simulink model "gm_HDL_pfc_gold_fi_og"  (R2024b)
settings: Solver=FixedStepDiscrete  StartTime=0.0  StopTime=.2  RelTol=1e-3
InitFcn:
  | fidelity_pfc_vals;
  | nbits=(2^12)-2;
  | A_mat = fi(stateSpaceParameters_1.Ad,1,25,24);
  | B_mat = fi(stateSpaceParameters_1.Bd,1,25,31);
  | C_mat = fi(stateSpaceParameters_1.Cd,1,25,20);
  | D_mat = fi(stateSpaceParameters_1.Dd,1,25,19);
  | X0_mat= fi(stateSpaceParameters_1.X0,1,25,14);
  | load('C:\Users\Angel\Desktop\hil\pfc3ph\matlab\sim\sschdl\pfc_desktop\stateSpaceParameters.mat');
undefined symbols (not defined in the file or in its folder): a, b, c, fsw, t_ss, tsw
libraries: simulink x39, hdlmdlgenlib x24, hdlsllib x9, mcbcontrolslib x5, dspsrcs4 x3, slpidlib x2, spsSVPWMGenerator2LevelLib x1, spsPLL3phLib x1, fillib x1
(part 3 of 4)

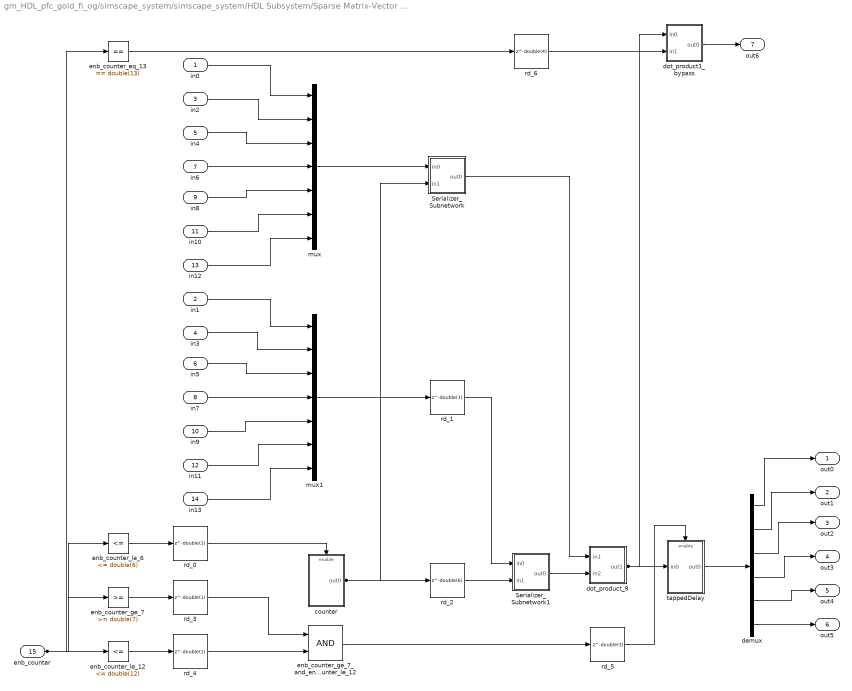
== system gm_HDL_pfc_gold_fi_og/simscape_system/simscape_system/HDL Subsystem/Sparse Matrix-Vector Product/hNNewMatrixB_shared ==
  in0 : Inport  OutDataTypeStr=fixdt(1, 25, 31)  PortDimensions=[9]  SampleTime=1.0465724751439e-08
  in1 : Inport  Port=2  OutDataTypeStr=fixdt(1, 25, 13)  PortDimensions=[9]  SampleTime=1.0465724751439e-08
  in2 : Inport  Port=3  OutDataTypeStr=fixdt(1, 25, 31)  PortDimensions=[9]  SampleTime=1.0465724751439e-08
  in3 : Inport  Port=4  OutDataTypeStr=fixdt(1, 25, 13)  PortDimensions=[9]  SampleTime=1.0465724751439e-08
  in4 : Inport  Port=5  OutDataTypeStr=fixdt(1, 25, 31)  PortDimensions=[9]  SampleTime=1.0465724751439e-08
  in5 : Inport  Port=6  OutDataTypeStr=fixdt(1, 25, 13)  PortDimensions=[9]  SampleTime=1.0465724751439e-08
  in6 : Inport  Port=7  OutDataTypeStr=fixdt(1, 25, 31)  PortDimensions=[9]  SampleTime=1.0465724751439e-08
  in7 : Inport  Port=8  OutDataTypeStr=fixdt(1, 25, 13)  PortDimensions=[9]  SampleTime=1.0465724751439e-08
  in8 : Inport  Port=9  OutDataTypeStr=fixdt(1, 25, 31)  PortDimensions=[9]  SampleTime=1.0465724751439e-08
  in9 : Inport  Port=10  OutDataTypeStr=fixdt(1, 25, 13)  PortDimensions=[9]  SampleTime=1.0465724751439e-08
  in10 : Inport  Port=11  OutDataTypeStr=fixdt(1, 25, 31)  PortDimensions=[9]  SampleTime=1.0465724751439e-08
  in11 : Inport  Port=12  OutDataTypeStr=fixdt(1, 25, 13)  PortDimensions=[9]  SampleTime=1.0465724751439e-08
  in12 : Inport  Port=13  OutDataTypeStr=fixdt(1, 25, 31)  PortDimensions=[9]  SampleTime=1.0465724751439e-08
  in13 : Inport  Port=14  OutDataTypeStr=fixdt(1, 25, 13)  PortDimensions=[9]  SampleTime=1.0465724751439e-08
  enb_counter : Inport  Port=15  OutDataTypeStr=fixdt(0, 6, 0)  SampleTime=1.0465724751439e-08
  Serializer_Subnetwork : Subsystem
  Serializer_Subnetwork1 : Subsystem
  counter : Subsystem
  demux : Demux  Outputs=6
  dot_product1_bypass : Subsystem
  dot_product_9 : Subsystem
  enb_counter_eq_13 : simulink/Logic and Bit Operations/Compare To Constant  relop===  const=double(13)  OutDataTypeStr=boolean
  enb_counter_ge_7 : simulink/Logic and Bit Operations/Compare To Constant  relop=>=  const=double(7)  OutDataTypeStr=boolean
  enb_counter_ge_7_and_enb_counter_le_12 : Logic  AllPortsSameDT=off  OutDataTypeStr=boolean  SampleTime=1.0465724751439e-08
  enb_counter_le_12 : simulink/Logic and Bit Operations/Compare To Constant  relop=<=  const=double(12)  OutDataTypeStr=boolean
  enb_counter_le_6 : simulink/Logic and Bit Operations/Compare To Constant  relop=<=  const=double(6)  OutDataTypeStr=boolean
  mux : Mux  Inputs=7
  mux1 : Mux  Inputs=7
  rd_{0..1,3..4} (4 alike) : Delay  DelayLength=double(1)  InitialCondition=0  SampleTime=1.0465724751439e-08
  rd_2 : Delay  DelayLength=double(6)  InitialCondition=0  SampleTime=1.0465724751439e-08
  rd_5 : Delay  DelayLength=double(3)  InitialCondition=0  SampleTime=1.0465724751439e-08
  rd_6 : Delay  DelayLength=double(4)  InitialCondition=0  SampleTime=1.0465724751439e-08
  tappedDelay : Subsystem
  out0 : Outport  OutDataTypeStr=fixdt(1, 50, 44)  SampleTime=1.0465724751439e-08
  out1 : Outport  Port=2  OutDataTypeStr=fixdt(1, 50, 44)  SampleTime=1.0465724751439e-08
  out2 : Outport  Port=3  OutDataTypeStr=fixdt(1, 50, 44)  SampleTime=1.0465724751439e-08
  out3 : Outport  Port=4  OutDataTypeStr=fixdt(1, 50, 44)  SampleTime=1.0465724751439e-08
  out4 : Outport  Port=5  OutDataTypeStr=fixdt(1, 50, 44)  SampleTime=1.0465724751439e-08
  out5 : Outport  Port=6  OutDataTypeStr=fixdt(1, 50, 44)  SampleTime=1.0465724751439e-08
  out6 : Outport  Port=7  OutDataTypeStr=fixdt(1, 50, 44)  SampleTime=1.0465724751439e-08
  wires:
  enb_counter_le_12/1 -> rd_4/1
  rd_1/1 -> Serializer_Subnetwork1/1(in0)
  enb_counter/1 -> enb_counter_le_12/1, enb_counter_ge_7/1, enb_counter_le_6/1, enb_counter_eq_13/1
  in4/1 -> mux/3
  rd_0/1 -> counter/Enable
  enb_counter_eq_13/1 -> rd_6/1
  demux/4 -> out3/1
  enb_counter_le_6/1 -> rd_0/1
  enb_counter_ge_7/1 -> rd_3/1
  demux/6 -> out5/1
  rd_3/1 -> enb_counter_ge_7_and_enb_counter_le_12/1
  in2/1 -> mux/2
  in0/1 -> mux/1
  in6/1 -> mux/4
  in8/1 -> mux/5
  in10/1 -> mux/6
  dot_product1_bypass/1(out0) -> out6/1
  in9/1 -> mux1/5
  in12/1 -> mux/7
  in1/1 -> mux1/1
  in3/1 -> mux1/2
  tappedDelay/1(out0) -> demux/1
  enb_counter_ge_7_and_enb_counter_le_12/1 -> rd_5/1
  in5/1 -> mux1/3
  in7/1 -> mux1/4
  in11/1 -> mux1/6
  dot_product_9/1(out1) -> dot_product1_bypass/1(in0), tappedDelay/1(in0)
  mux/1 -> Serializer_Subnetwork/1(in0)
  in13/1 -> mux1/7
  demux/3 -> out2/1
  rd_4/1 -> enb_counter_ge_7_and_enb_counter_le_12/2
  Serializer_Subnetwork/1(out0) -> dot_product_9/1(in1)
  mux1/1 -> rd_1/1
  counter/1(out0) -> rd_2/1, Serializer_Subnetwork/2(in1)
  rd_2/1 -> Serializer_Subnetwork1/2(in1)
  rd_6/1 -> dot_product1_bypass/2(in1)
  Serializer_Subnetwork1/1(out0) -> dot_product_9/2(in2)
  rd_5/1 -> tappedDelay/Enable
  demux/5 -> out4/1
  demux/1 -> out0/1
  demux/2 -> out1/1

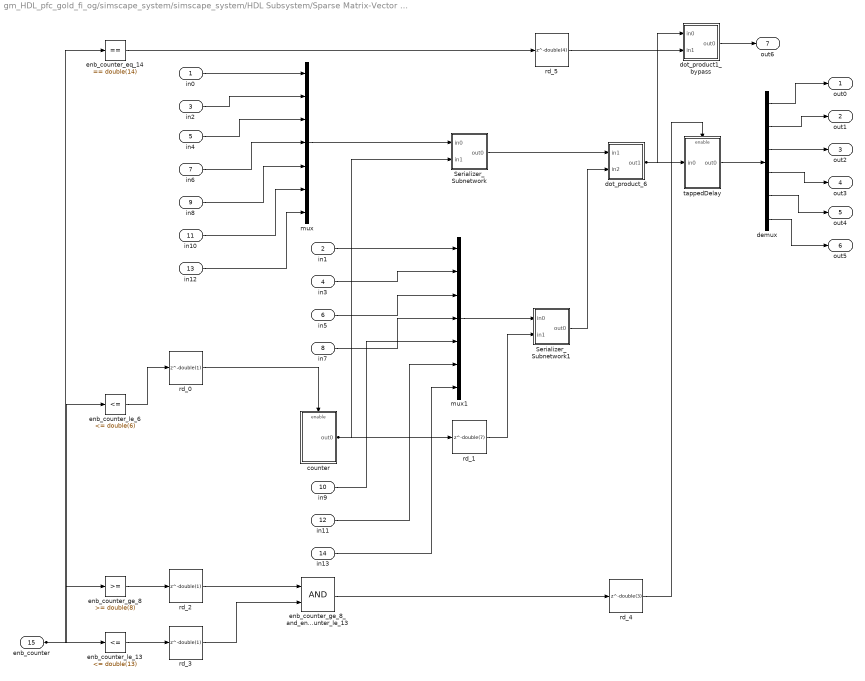
== system gm_HDL_pfc_gold_fi_og/simscape_system/simscape_system/HDL Subsystem/Sparse Matrix-Vector Product1/hNNewMatrixA_shared ==
  in0 : Inport  OutDataTypeStr=fixdt(1, 25, 24)  PortDimensions=[6]  SampleTime=1.0465724751439e-08
  in1 : Inport  Port=2  OutDataTypeStr=fixdt(1, 25, 13)  PortDimensions=[6]  SampleTime=1.0465724751439e-08
  in2 : Inport  Port=3  OutDataTypeStr=fixdt(1, 25, 24)  PortDimensions=[6]  SampleTime=1.0465724751439e-08
  in3 : Inport  Port=4  OutDataTypeStr=fixdt(1, 25, 13)  PortDimensions=[6]  SampleTime=1.0465724751439e-08
  in4 : Inport  Port=5  OutDataTypeStr=fixdt(1, 25, 24)  PortDimensions=[6]  SampleTime=1.0465724751439e-08
  in5 : Inport  Port=6  OutDataTypeStr=fixdt(1, 25, 13)  PortDimensions=[6]  SampleTime=1.0465724751439e-08
  in6 : Inport  Port=7  OutDataTypeStr=fixdt(1, 25, 24)  PortDimensions=[6]  SampleTime=1.0465724751439e-08
  in7 : Inport  Port=8  OutDataTypeStr=fixdt(1, 25, 13)  PortDimensions=[6]  SampleTime=1.0465724751439e-08
  in8 : Inport  Port=9  OutDataTypeStr=fixdt(1, 25, 24)  PortDimensions=[6]  SampleTime=1.0465724751439e-08
  in9 : Inport  Port=10  OutDataTypeStr=fixdt(1, 25, 13)  PortDimensions=[6]  SampleTime=1.0465724751439e-08
  in10 : Inport  Port=11  OutDataTypeStr=fixdt(1, 25, 24)  PortDimensions=[6]  SampleTime=1.0465724751439e-08
  in11 : Inport  Port=12  OutDataTypeStr=fixdt(1, 25, 13)  PortDimensions=[6]  SampleTime=1.0465724751439e-08
  in12 : Inport  Port=13  OutDataTypeStr=fixdt(1, 25, 24)  PortDimensions=[6]  SampleTime=1.0465724751439e-08
  in13 : Inport  Port=14  OutDataTypeStr=fixdt(1, 25, 13)  PortDimensions=[6]  SampleTime=1.0465724751439e-08
  enb_counter : Inport  Port=15  OutDataTypeStr=fixdt(0, 6, 0)  SampleTime=1.0465724751439e-08
  Serializer_Subnetwork : Subsystem
  Serializer_Subnetwork1 : Subsystem
  counter : Subsystem
  demux : Demux  Outputs=6
  dot_product1_bypass : Subsystem
  dot_product_6 : Subsystem
  enb_counter_eq_14 : simulink/Logic and Bit Operations/Compare To Constant  relop===  const=double(14)  OutDataTypeStr=boolean
  enb_counter_ge_8 : simulink/Logic and Bit Operations/Compare To Constant  relop=>=  const=double(8)  OutDataTypeStr=boolean
  enb_counter_ge_8_and_enb_counter_le_13 : Logic  AllPortsSameDT=off  OutDataTypeStr=boolean  SampleTime=1.0465724751439e-08
  enb_counter_le_13 : simulink/Logic and Bit Operations/Compare To Constant  relop=<=  const=double(13)  OutDataTypeStr=boolean
  enb_counter_le_6 : simulink/Logic and Bit Operations/Compare To Constant  relop=<=  const=double(6)  OutDataTypeStr=boolean
  mux : Mux  Inputs=7
  mux1 : Mux  Inputs=7
  rd_0 : Delay  DelayLength=double(1)  InitialCondition=0  SampleTime=1.0465724751439e-08
  rd_1 : Delay  DelayLength=double(7)  InitialCondition=0  SampleTime=1.0465724751439e-08
  rd_2 : Delay  DelayLength=double(1)  InitialCondition=0  SampleTime=1.0465724751439e-08
  rd_3 : Delay  DelayLength=double(1)  InitialCondition=0  SampleTime=1.0465724751439e-08
  rd_4 : Delay  DelayLength=double(3)  InitialCondition=0  SampleTime=1.0465724751439e-08
  rd_5 : Delay  DelayLength=double(4)  InitialCondition=0  SampleTime=1.0465724751439e-08
  tappedDelay : Subsystem
  out0 : Outport  OutDataTypeStr=fixdt(1, 50, 37)  SampleTime=1.0465724751439e-08
  out1 : Outport  Port=2  OutDataTypeStr=fixdt(1, 50, 37)  SampleTime=1.0465724751439e-08
  out2 : Outport  Port=3  OutDataTypeStr=fixdt(1, 50, 37)  SampleTime=1.0465724751439e-08
  out3 : Outport  Port=4  OutDataTypeStr=fixdt(1, 50, 37)  SampleTime=1.0465724751439e-08
  out4 : Outport  Port=5  OutDataTypeStr=fixdt(1, 50, 37)  SampleTime=1.0465724751439e-08
  out5 : Outport  Port=6  OutDataTypeStr=fixdt(1, 50, 37)  SampleTime=1.0465724751439e-08
  out6 : Outport  Port=7  OutDataTypeStr=fixdt(1, 50, 37)  SampleTime=1.0465724751439e-08
  wires:
  rd_0/1 -> counter/Enable
  in0/1 -> mux/1
  Serializer_Subnetwork/1(out0) -> dot_product_6/1(in1)
  enb_counter/1 -> enb_counter_ge_8/1, enb_counter_le_6/1, enb_counter_le_13/1, enb_counter_eq_14/1
  enb_counter_eq_14/1 -> rd_5/1
  demux/6 -> out5/1
  in4/1 -> mux/3
  enb_counter_le_13/1 -> rd_3/1
  enb_counter_le_6/1 -> rd_0/1
  mux/1 -> Serializer_Subnetwork/1(in0)
  enb_counter_ge_8/1 -> rd_2/1
  in1/1 -> mux1/1
  in2/1 -> mux/2
  in6/1 -> mux/4
  enb_counter_ge_8_and_enb_counter_le_13/1 -> rd_4/1
  in8/1 -> mux/5
  in10/1 -> mux/6
  demux/2 -> out1/1
  in12/1 -> mux/7
  rd_2/1 -> enb_counter_ge_8_and_enb_counter_le_13/1
  Serializer_Subnetwork1/1(out0) -> dot_product_6/2(in2)
  rd_3/1 -> enb_counter_ge_8_and_enb_counter_le_13/2
  demux/5 -> out4/1
  in3/1 -> mux1/2
  in5/1 -> mux1/3
  tappedDelay/1(out0) -> demux/1
  in7/1 -> mux1/4
  counter/1(out0) -> rd_1/1, Serializer_Subnetwork/2(in1)
  in9/1 -> mux1/5
  in11/1 -> mux1/6
  in13/1 -> mux1/7
  mux1/1 -> Serializer_Subnetwork1/1(in0)
  dot_product_6/1(out1) -> tappedDelay/1(in0), dot_product1_bypass/1(in0)
  rd_1/1 -> Serializer_Subnetwork1/2(in1)
  rd_5/1 -> dot_product1_bypass/2(in1)
  rd_4/1 -> tappedDelay/Enable
  dot_product1_bypass/1(out0) -> out6/1
  demux/1 -> out0/1
  demux/3 -> out2/1
  demux/4 -> out3/1

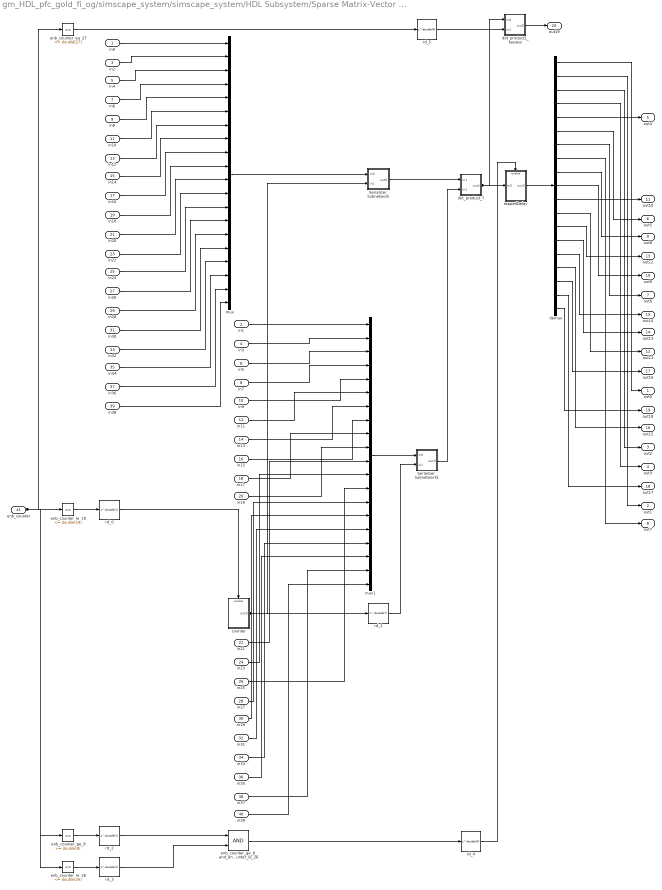
== system gm_HDL_pfc_gold_fi_og/simscape_system/simscape_system/HDL Subsystem/Sparse Matrix-Vector Product2/hNNewMatrixC_shared ==
  in0 : Inport  OutDataTypeStr=fixdt(1, 25, 20)  PortDimensions=[7]  SampleTime=1.0465724751439e-08
  in1 : Inport  Port=2  OutDataTypeStr=fixdt(1, 25, 13)  PortDimensions=[7]  SampleTime=1.0465724751439e-08
  in2 : Inport  Port=3  OutDataTypeStr=fixdt(1, 25, 20)  PortDimensions=[7]  SampleTime=1.0465724751439e-08
  in3 : Inport  Port=4  OutDataTypeStr=fixdt(1, 25, 13)  PortDimensions=[7]  SampleTime=1.0465724751439e-08
  in4 : Inport  Port=5  OutDataTypeStr=fixdt(1, 25, 20)  PortDimensions=[7]  SampleTime=1.0465724751439e-08
  in5 : Inport  Port=6  OutDataTypeStr=fixdt(1, 25, 13)  PortDimensions=[7]  SampleTime=1.0465724751439e-08
  in6 : Inport  Port=7  OutDataTypeStr=fixdt(1, 25, 20)  PortDimensions=[7]  SampleTime=1.0465724751439e-08
  in7 : Inport  Port=8  OutDataTypeStr=fixdt(1, 25, 13)  PortDimensions=[7]  SampleTime=1.0465724751439e-08
  in8 : Inport  Port=9  OutDataTypeStr=fixdt(1, 25, 20)  PortDimensions=[7]  SampleTime=1.0465724751439e-08
  in9 : Inport  Port=10  OutDataTypeStr=fixdt(1, 25, 13)  PortDimensions=[7]  SampleTime=1.0465724751439e-08
  in10 : Inport  Port=11  OutDataTypeStr=fixdt(1, 25, 20)  PortDimensions=[7]  SampleTime=1.0465724751439e-08
  in11 : Inport  Port=12  OutDataTypeStr=fixdt(1, 25, 13)  PortDimensions=[7]  SampleTime=1.0465724751439e-08
  in12 : Inport  Port=13  OutDataTypeStr=fixdt(1, 25, 20)  PortDimensions=[7]  SampleTime=1.0465724751439e-08
  in13 : Inport  Port=14  OutDataTypeStr=fixdt(1, 25, 13)  PortDimensions=[7]  SampleTime=1.0465724751439e-08
  in14 : Inport  Port=15  OutDataTypeStr=fixdt(1, 25, 20)  PortDimensions=[7]  SampleTime=1.0465724751439e-08
  in15 : Inport  Port=16  OutDataTypeStr=fixdt(1, 25, 13)  PortDimensions=[7]  SampleTime=1.0465724751439e-08
  in16 : Inport  Port=17  OutDataTypeStr=fixdt(1, 25, 20)  PortDimensions=[7]  SampleTime=1.0465724751439e-08
  in17 : Inport  Port=18  OutDataTypeStr=fixdt(1, 25, 13)  PortDimensions=[7]  SampleTime=1.0465724751439e-08
  in18 : Inport  Port=19  OutDataTypeStr=fixdt(1, 25, 20)  PortDimensions=[7]  SampleTime=1.0465724751439e-08
  in19 : Inport  Port=20  OutDataTypeStr=fixdt(1, 25, 13)  PortDimensions=[7]  SampleTime=1.0465724751439e-08
  in20 : Inport  Port=21  OutDataTypeStr=fixdt(1, 25, 20)  PortDimensions=[7]  SampleTime=1.0465724751439e-08
  in21 : Inport  Port=22  OutDataTypeStr=fixdt(1, 25, 13)  PortDimensions=[7]  SampleTime=1.0465724751439e-08
  in22 : Inport  Port=23  OutDataTypeStr=fixdt(1, 25, 20)  PortDimensions=[7]  SampleTime=1.0465724751439e-08
  in23 : Inport  Port=24  OutDataTypeStr=fixdt(1, 25, 13)  PortDimensions=[7]  SampleTime=1.0465724751439e-08
  in24 : Inport  Port=25  OutDataTypeStr=fixdt(1, 25, 20)  PortDimensions=[7]  SampleTime=1.0465724751439e-08
  in25 : Inport  Port=26  OutDataTypeStr=fixdt(1, 25, 13)  PortDimensions=[7]  SampleTime=1.0465724751439e-08
  in26 : Inport  Port=27  OutDataTypeStr=fixdt(1, 25, 20)  PortDimensions=[7]  SampleTime=1.0465724751439e-08
  in27 : Inport  Port=28  OutDataTypeStr=fixdt(1, 25, 13)  PortDimensions=[7]  SampleTime=1.0465724751439e-08
  in28 : Inport  Port=29  OutDataTypeStr=fixdt(1, 25, 20)  PortDimensions=[7]  SampleTime=1.0465724751439e-08
  in29 : Inport  Port=30  OutDataTypeStr=fixdt(1, 25, 13)  PortDimensions=[7]  SampleTime=1.0465724751439e-08
  in30 : Inport  Port=31  OutDataTypeStr=fixdt(1, 25, 20)  PortDimensions=[7]  SampleTime=1.0465724751439e-08
  in31 : Inport  Port=32  OutDataTypeStr=fixdt(1, 25, 13)  PortDimensions=[7]  SampleTime=1.0465724751439e-08
  in32 : Inport  Port=33  OutDataTypeStr=fixdt(1, 25, 20)  PortDimensions=[7]  SampleTime=1.0465724751439e-08
  in33 : Inport  Port=34  OutDataTypeStr=fixdt(1, 25, 13)  PortDimensions=[7]  SampleTime=1.0465724751439e-08
  in34 : Inport  Port=35  OutDataTypeStr=fixdt(1, 25, 20)  PortDimensions=[7]  SampleTime=1.0465724751439e-08
  in35 : Inport  Port=36  OutDataTypeStr=fixdt(1, 25, 13)  PortDimensions=[7]  SampleTime=1.0465724751439e-08
  in36 : Inport  Port=37  OutDataTypeStr=fixdt(1, 25, 20)  PortDimensions=[7]  SampleTime=1.0465724751439e-08
  in37 : Inport  Port=38  OutDataTypeStr=fixdt(1, 25, 13)  PortDimensions=[7]  SampleTime=1.0465724751439e-08
  in38 : Inport  Port=39  OutDataTypeStr=fixdt(1, 25, 20)  PortDimensions=[7]  SampleTime=1.0465724751439e-08
  in39 : Inport  Port=40  OutDataTypeStr=fixdt(1, 25, 13)  PortDimensions=[7]  SampleTime=1.0465724751439e-08
  enb_counter : Inport  Port=41  OutDataTypeStr=fixdt(0, 6, 0)  SampleTime=1.0465724751439e-08
  Serializer_Subnetwork : Subsystem
  Serializer_Subnetwork1 : Subsystem
  counter : Subsystem
  demux : Demux  Outputs=19
  dot_product1_bypass : Subsystem
  dot_product_7 : Subsystem
  enb_counter_eq_27 : simulink/Logic and Bit Operations/Compare To Constant  relop===  const=double(27)  OutDataTypeStr=boolean
  enb_counter_ge_8 : simulink/Logic and Bit Operations/Compare To Constant  relop=>=  const=double(8)  OutDataTypeStr=boolean
  enb_counter_ge_8_and_enb_counter_le_26 : Logic  AllPortsSameDT=off  OutDataTypeStr=boolean  SampleTime=1.0465724751439e-08
  enb_counter_le_19 : simulink/Logic and Bit Operations/Compare To Constant  relop=<=  const=double(19)  OutDataTypeStr=boolean
  enb_counter_le_26 : simulink/Logic and Bit Operations/Compare To Constant  relop=<=  const=double(26)  OutDataTypeStr=boolean
  mux : Mux  Inputs=20
  mux1 : Mux  Inputs=20
  rd_0 : Delay  DelayLength=double(1)  InitialCondition=0  SampleTime=1.0465724751439e-08
  rd_1 : Delay  DelayLength=double(7)  InitialCondition=0  SampleTime=1.0465724751439e-08
  rd_2 : Delay  DelayLength=double(1)  InitialCondition=0  SampleTime=1.0465724751439e-08
  rd_3 : Delay  DelayLength=double(1)  InitialCondition=0  SampleTime=1.0465724751439e-08
  rd_4 : Delay  DelayLength=double(3)  InitialCondition=0  SampleTime=1.0465724751439e-08
  rd_5 : Delay  DelayLength=double(4)  InitialCondition=0  SampleTime=1.0465724751439e-08
  tappedDelay : Subsystem
  out0 : Outport  OutDataTypeStr=fixdt(1, 50, 33)  SampleTime=1.0465724751439e-08
  out1 : Outport  Port=2  OutDataTypeStr=fixdt(1, 50, 33)  SampleTime=1.0465724751439e-08
  out2 : Outport  Port=3  OutDataTypeStr=fixdt(1, 50, 33)  SampleTime=1.0465724751439e-08
  out3 : Outport  Port=4  OutDataTypeStr=fixdt(1, 50, 33)  SampleTime=1.0465724751439e-08
  out4 : Outport  Port=5  OutDataTypeStr=fixdt(1, 50, 33)  SampleTime=1.0465724751439e-08
  out5 : Outport  Port=6  OutDataTypeStr=fixdt(1, 50, 33)  SampleTime=1.0465724751439e-08
  out6 : Outport  Port=7  OutDataTypeStr=fixdt(1, 50, 33)  SampleTime=1.0465724751439e-08
  out7 : Outport  Port=8  OutDataTypeStr=fixdt(1, 50, 33)  SampleTime=1.0465724751439e-08
  out8 : Outport  Port=9  OutDataTypeStr=fixdt(1, 50, 33)  SampleTime=1.0465724751439e-08
  out9 : Outport  Port=10  OutDataTypeStr=fixdt(1, 50, 33)  SampleTime=1.0465724751439e-08
  out10 : Outport  Port=11  OutDataTypeStr=fixdt(1, 50, 33)  SampleTime=1.0465724751439e-08
  out11 : Outport  Port=12  OutDataTypeStr=fixdt(1, 50, 33)  SampleTime=1.0465724751439e-08
  out12 : Outport  Port=13  OutDataTypeStr=fixdt(1, 50, 33)  SampleTime=1.0465724751439e-08
  out13 : Outport  Port=14  OutDataTypeStr=fixdt(1, 50, 33)  SampleTime=1.0465724751439e-08
  out14 : Outport  Port=15  OutDataTypeStr=fixdt(1, 50, 33)  SampleTime=1.0465724751439e-08
  out15 : Outport  Port=16  OutDataTypeStr=fixdt(1, 50, 33)  SampleTime=1.0465724751439e-08
  out16 : Outport  Port=17  OutDataTypeStr=fixdt(1, 50, 33)  SampleTime=1.0465724751439e-08
  out17 : Outport  Port=18  OutDataTypeStr=fixdt(1, 50, 33)  SampleTime=1.0465724751439e-08
  out18 : Outport  Port=19  OutDataTypeStr=fixdt(1, 50, 33)  SampleTime=1.0465724751439e-08
  out19 : Outport  Port=20  OutDataTypeStr=fixdt(1, 50, 33)  SampleTime=1.0465724751439e-08
  wires:
  enb_counter_le_19/1 -> rd_0/1
  enb_counter/1 -> enb_counter_le_26/1, enb_counter_ge_8/1, enb_counter_le_19/1, enb_counter_eq_27/1
  in29/1 -> mux1/15
  in27/1 -> mux1/14
  enb_counter_eq_27/1 -> rd_5/1
  rd_1/1 -> Serializer_Subnetwork1/2(in1)
  in4/1 -> mux/3
  in24/1 -> mux/13
  in0/1 -> mux/1
  enb_counter_ge_8/1 -> rd_2/1
  in5/1 -> mux1/3
  enb_counter_le_26/1 -> rd_3/1
  tappedDelay/1(out0) -> demux/1
  in2/1 -> mux/2
  in38/1 -> mux/20
  in8/1 -> mux/5
  in6/1 -> mux/4
  in10/1 -> mux/6
  in12/1 -> mux/7
  in16/1 -> mux/9
  in14/1 -> mux/8
  in18/1 -> mux/10
  in20/1 -> mux/11
  in22/1 -> mux/12
  in26/1 -> mux/14
  rd_0/1 -> counter/Enable
  demux/9 -> out8/1
  in28/1 -> mux/15
  in32/1 -> mux/17
  demux/19 -> out18/1
  in30/1 -> mux/16
  in1/1 -> mux1/1
  in34/1 -> mux/18
  rd_4/1 -> tappedDelay/Enable
  in36/1 -> mux/19
  counter/1(out0) -> Serializer_Subnetwork/2(in1), rd_1/1
  rd_2/1 -> enb_counter_ge_8_and_enb_counter_le_26/1
  rd_3/1 -> enb_counter_ge_8_and_enb_counter_le_26/2
  mux/1 -> Serializer_Subnetwork/1(in0)
  in3/1 -> mux1/2
  in7/1 -> mux1/4
  in9/1 -> mux1/5
  in13/1 -> mux1/7
  in11/1 -> mux1/6
  in15/1 -> mux1/8
  in17/1 -> mux1/9
  in21/1 -> mux1/11
  in19/1 -> mux1/10
  in23/1 -> mux1/12
  in25/1 -> mux1/13
  in31/1 -> mux1/16
  Serializer_Subnetwork/1(out0) -> dot_product_7/1(in1)
  in33/1 -> mux1/17
  in35/1 -> mux1/18
  in37/1 -> mux1/19
  in39/1 -> mux1/20
  enb_counter_ge_8_and_enb_counter_le_26/1 -> rd_4/1
  mux1/1 -> Serializer_Subnetwork1/1(in0)
  rd_5/1 -> dot_product1_bypass/2(in1)
  demux/4 -> out3/1
  demux/2 -> out1/1
  demux/6 -> out5/1
  Serializer_Subnetwork1/1(out0) -> dot_product_7/2(in2)
  dot_product_7/1(out1) -> tappedDelay/1(in0), dot_product1_bypass/1(in0)
  dot_product1_bypass/1(out0) -> out19/1
  demux/3 -> out2/1
  demux/1 -> out0/1
  demux/5 -> out4/1
  demux/7 -> out6/1
  demux/8 -> out7/1
  demux/10 -> out9/1
  demux/11 -> out10/1
  demux/12 -> out11/1
  demux/13 -> out12/1
  demux/14 -> out13/1
  demux/15 -> out14/1
  demux/16 -> out15/1
  demux/17 -> out16/1
  demux/18 -> out17/1

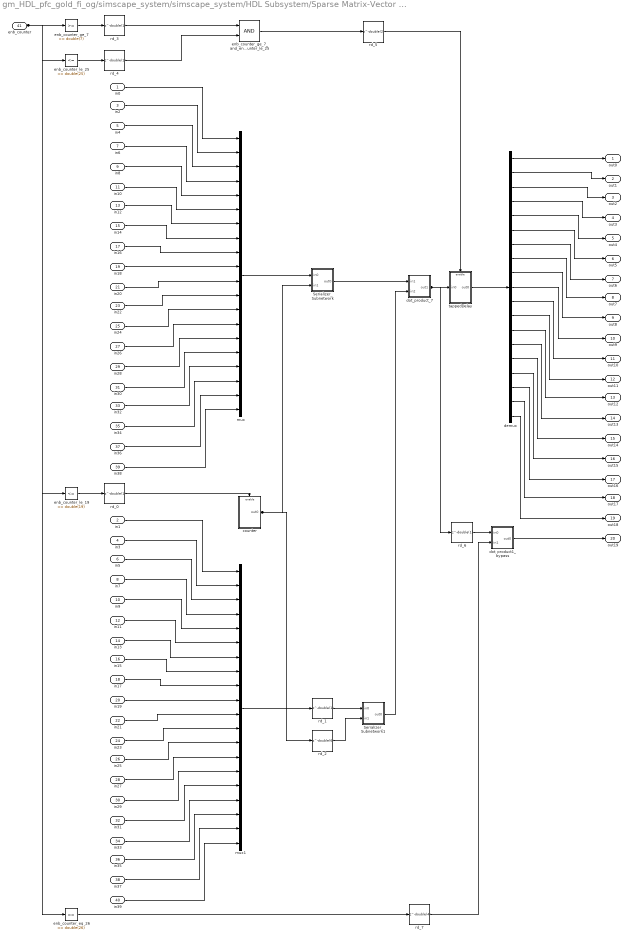
== system gm_HDL_pfc_gold_fi_og/simscape_system/simscape_system/HDL Subsystem/Sparse Matrix-Vector Product3/hNNewMatrixD_shared ==
  in0 : Inport  OutDataTypeStr=fixdt(1, 25, 19)  PortDimensions=[7]  SampleTime=1.0465724751439e-08
  in1 : Inport  Port=2  OutDataTypeStr=fixdt(1, 25, 13)  PortDimensions=[7]  SampleTime=1.0465724751439e-08
  in2 : Inport  Port=3  OutDataTypeStr=fixdt(1, 25, 19)  PortDimensions=[7]  SampleTime=1.0465724751439e-08
  in3 : Inport  Port=4  OutDataTypeStr=fixdt(1, 25, 13)  PortDimensions=[7]  SampleTime=1.0465724751439e-08
  in4 : Inport  Port=5  OutDataTypeStr=fixdt(1, 25, 19)  PortDimensions=[7]  SampleTime=1.0465724751439e-08
  in5 : Inport  Port=6  OutDataTypeStr=fixdt(1, 25, 13)  PortDimensions=[7]  SampleTime=1.0465724751439e-08
  in6 : Inport  Port=7  OutDataTypeStr=fixdt(1, 25, 19)  PortDimensions=[7]  SampleTime=1.0465724751439e-08
  in7 : Inport  Port=8  OutDataTypeStr=fixdt(1, 25, 13)  PortDimensions=[7]  SampleTime=1.0465724751439e-08
  in8 : Inport  Port=9  OutDataTypeStr=fixdt(1, 25, 19)  PortDimensions=[7]  SampleTime=1.0465724751439e-08
  in9 : Inport  Port=10  OutDataTypeStr=fixdt(1, 25, 13)  PortDimensions=[7]  SampleTime=1.0465724751439e-08
  in10 : Inport  Port=11  OutDataTypeStr=fixdt(1, 25, 19)  PortDimensions=[7]  SampleTime=1.0465724751439e-08
  in11 : Inport  Port=12  OutDataTypeStr=fixdt(1, 25, 13)  PortDimensions=[7]  SampleTime=1.0465724751439e-08
  in12 : Inport  Port=13  OutDataTypeStr=fixdt(1, 25, 19)  PortDimensions=[7]  SampleTime=1.0465724751439e-08
  in13 : Inport  Port=14  OutDataTypeStr=fixdt(1, 25, 13)  PortDimensions=[7]  SampleTime=1.0465724751439e-08
  in14 : Inport  Port=15  OutDataTypeStr=fixdt(1, 25, 19)  PortDimensions=[7]  SampleTime=1.0465724751439e-08
  in15 : Inport  Port=16  OutDataTypeStr=fixdt(1, 25, 13)  PortDimensions=[7]  SampleTime=1.0465724751439e-08
  in16 : Inport  Port=17  OutDataTypeStr=fixdt(1, 25, 19)  PortDimensions=[7]  SampleTime=1.0465724751439e-08
  in17 : Inport  Port=18  OutDataTypeStr=fixdt(1, 25, 13)  PortDimensions=[7]  SampleTime=1.0465724751439e-08
  in18 : Inport  Port=19  OutDataTypeStr=fixdt(1, 25, 19)  PortDimensions=[7]  SampleTime=1.0465724751439e-08
  in19 : Inport  Port=20  OutDataTypeStr=fixdt(1, 25, 13)  PortDimensions=[7]  SampleTime=1.0465724751439e-08
  in20 : Inport  Port=21  OutDataTypeStr=fixdt(1, 25, 19)  PortDimensions=[7]  SampleTime=1.0465724751439e-08
  in21 : Inport  Port=22  OutDataTypeStr=fixdt(1, 25, 13)  PortDimensions=[7]  SampleTime=1.0465724751439e-08
  in22 : Inport  Port=23  OutDataTypeStr=fixdt(1, 25, 19)  PortDimensions=[7]  SampleTime=1.0465724751439e-08
  in23 : Inport  Port=24  OutDataTypeStr=fixdt(1, 25, 13)  PortDimensions=[7]  SampleTime=1.0465724751439e-08
  in24 : Inport  Port=25  OutDataTypeStr=fixdt(1, 25, 19)  PortDimensions=[7]  SampleTime=1.0465724751439e-08
  in25 : Inport  Port=26  OutDataTypeStr=fixdt(1, 25, 13)  PortDimensions=[7]  SampleTime=1.0465724751439e-08
  in26 : Inport  Port=27  OutDataTypeStr=fixdt(1, 25, 19)  PortDimensions=[7]  SampleTime=1.0465724751439e-08
  in27 : Inport  Port=28  OutDataTypeStr=fixdt(1, 25, 13)  PortDimensions=[7]  SampleTime=1.0465724751439e-08
  in28 : Inport  Port=29  OutDataTypeStr=fixdt(1, 25, 19)  PortDimensions=[7]  SampleTime=1.0465724751439e-08
  in29 : Inport  Port=30  OutDataTypeStr=fixdt(1, 25, 13)  PortDimensions=[7]  SampleTime=1.0465724751439e-08
  in30 : Inport  Port=31  OutDataTypeStr=fixdt(1, 25, 19)  PortDimensions=[7]  SampleTime=1.0465724751439e-08
  in31 : Inport  Port=32  OutDataTypeStr=fixdt(1, 25, 13)  PortDimensions=[7]  SampleTime=1.0465724751439e-08
  in32 : Inport  Port=33  OutDataTypeStr=fixdt(1, 25, 19)  PortDimensions=[7]  SampleTime=1.0465724751439e-08
  in33 : Inport  Port=34  OutDataTypeStr=fixdt(1, 25, 13)  PortDimensions=[7]  SampleTime=1.0465724751439e-08
  in34 : Inport  Port=35  OutDataTypeStr=fixdt(1, 25, 19)  PortDimensions=[7]  SampleTime=1.0465724751439e-08
  in35 : Inport  Port=36  OutDataTypeStr=fixdt(1, 25, 13)  PortDimensions=[7]  SampleTime=1.0465724751439e-08
  in36 : Inport  Port=37  OutDataTypeStr=fixdt(1, 25, 19)  PortDimensions=[7]  SampleTime=1.0465724751439e-08
  in37 : Inport  Port=38  OutDataTypeStr=fixdt(1, 25, 13)  PortDimensions=[7]  SampleTime=1.0465724751439e-08
  in38 : Inport  Port=39  OutDataTypeStr=fixdt(1, 25, 19)  PortDimensions=[7]  SampleTime=1.0465724751439e-08
  in39 : Inport  Port=40  OutDataTypeStr=fixdt(1, 25, 13)  PortDimensions=[7]  SampleTime=1.0465724751439e-08
  enb_counter : Inport  Port=41  OutDataTypeStr=fixdt(0, 6, 0)  SampleTime=1.0465724751439e-08
  Serializer_Subnetwork : Subsystem
  Serializer_Subnetwork1 : Subsystem
  counter : Subsystem
  demux : Demux  Outputs=19
  dot_product1_bypass : Subsystem
  dot_product_7 : Subsystem
  enb_counter_eq_26 : simulink/Logic and Bit Operations/Compare To Constant  relop===  const=double(26)  OutDataTypeStr=boolean
  enb_counter_ge_7 : simulink/Logic and Bit Operations/Compare To Constant  relop=>=  const=double(7)  OutDataTypeStr=boolean
  enb_counter_ge_7_and_enb_counter_le_25 : Logic  AllPortsSameDT=off  OutDataTypeStr=boolean  SampleTime=1.0465724751439e-08
  enb_counter_le_19 : simulink/Logic and Bit Operations/Compare To Constant  relop=<=  const=double(19)  OutDataTypeStr=boolean
  enb_counter_le_25 : simulink/Logic and Bit Operations/Compare To Constant  relop=<=  const=double(25)  OutDataTypeStr=boolean
  mux : Mux  Inputs=20
  mux1 : Mux  Inputs=20
  rd_{0..1,3..4,6} (5 alike) : Delay  DelayLength=double(1)  InitialCondition=0  SampleTime=1.0465724751439e-08
  rd_2 : Delay  DelayLength=double(6)  InitialCondition=0  SampleTime=1.0465724751439e-08
  rd_5 : Delay  DelayLength=double(2)  InitialCondition=0  SampleTime=1.0465724751439e-08
  rd_7 : Delay  DelayLength=double(4)  InitialCondition=0  SampleTime=1.0465724751439e-08
  tappedDelay : Subsystem
  out0 : Outport  OutDataTypeStr=fixdt(1, 50, 32)  SampleTime=1.0465724751439e-08
  out1 : Outport  Port=2  OutDataTypeStr=fixdt(1, 50, 32)  SampleTime=1.0465724751439e-08
  out2 : Outport  Port=3  OutDataTypeStr=fixdt(1, 50, 32)  SampleTime=1.0465724751439e-08
  out3 : Outport  Port=4  OutDataTypeStr=fixdt(1, 50, 32)  SampleTime=1.0465724751439e-08
  out4 : Outport  Port=5  OutDataTypeStr=fixdt(1, 50, 32)  SampleTime=1.0465724751439e-08
  out5 : Outport  Port=6  OutDataTypeStr=fixdt(1, 50, 32)  SampleTime=1.0465724751439e-08
  out6 : Outport  Port=7  OutDataTypeStr=fixdt(1, 50, 32)  SampleTime=1.0465724751439e-08
  out7 : Outport  Port=8  OutDataTypeStr=fixdt(1, 50, 32)  SampleTime=1.0465724751439e-08
  out8 : Outport  Port=9  OutDataTypeStr=fixdt(1, 50, 32)  SampleTime=1.0465724751439e-08
  out9 : Outport  Port=10  OutDataTypeStr=fixdt(1, 50, 32)  SampleTime=1.0465724751439e-08
  out10 : Outport  Port=11  OutDataTypeStr=fixdt(1, 50, 32)  SampleTime=1.0465724751439e-08
  out11 : Outport  Port=12  OutDataTypeStr=fixdt(1, 50, 32)  SampleTime=1.0465724751439e-08
  out12 : Outport  Port=13  OutDataTypeStr=fixdt(1, 50, 32)  SampleTime=1.0465724751439e-08
  out13 : Outport  Port=14  OutDataTypeStr=fixdt(1, 50, 32)  SampleTime=1.0465724751439e-08
  out14 : Outport  Port=15  OutDataTypeStr=fixdt(1, 50, 32)  SampleTime=1.0465724751439e-08
  out15 : Outport  Port=16  OutDataTypeStr=fixdt(1, 50, 32)  SampleTime=1.0465724751439e-08
  out16 : Outport  Port=17  OutDataTypeStr=fixdt(1, 50, 32)  SampleTime=1.0465724751439e-08
  out17 : Outport  Port=18  OutDataTypeStr=fixdt(1, 50, 32)  SampleTime=1.0465724751439e-08
  out18 : Outport  Port=19  OutDataTypeStr=fixdt(1, 50, 32)  SampleTime=1.0465724751439e-08
  out19 : Outport  Port=20  OutDataTypeStr=fixdt(1, 50, 32)  SampleTime=1.0465724751439e-08
  wires:
  enb_counter/1 -> enb_counter_eq_26/1, enb_counter_ge_7/1, enb_counter_le_19/1, enb_counter_le_25/1
  enb_counter_eq_26/1 -> rd_7/1
  enb_counter_le_25/1 -> rd_4/1
  enb_counter_ge_7/1 -> rd_3/1
  in33/1 -> mux1/17
  in31/1 -> mux1/16
  rd_3/1 -> enb_counter_ge_7_and_enb_counter_le_25/1
  in16/1 -> mux/9
  enb_counter_le_19/1 -> rd_0/1
  in8/1 -> mux/5
  rd_4/1 -> enb_counter_ge_7_and_enb_counter_le_25/2
  tappedDelay/1(out0) -> demux/1
  in0/1 -> mux/1
  in36/1 -> mux/19
  in2/1 -> mux/2
  in23/1 -> mux1/12
  in4/1 -> mux/3
  in25/1 -> mux1/13
  in18/1 -> mux/10
  in6/1 -> mux/4
  rd_0/1 -> counter/Enable
  in10/1 -> mux/6
  demux/9 -> out8/1
  in12/1 -> mux/7
  in14/1 -> mux/8
  in20/1 -> mux/11
  in13/1 -> mux1/7
  in22/1 -> mux/12
  in30/1 -> mux/16
  rd_6/1 -> dot_product1_bypass/1(in0)
  in24/1 -> mux/13
  in37/1 -> mux1/19
  in26/1 -> mux/14
  in28/1 -> mux/15
  enb_counter_ge_7_and_enb_counter_le_25/1 -> rd_5/1
  in32/1 -> mux/17
  in34/1 -> mux/18
  in17/1 -> mux1/9
  demux/2 -> out1/1
  in38/1 -> mux/20
  in1/1 -> mux1/1
  in3/1 -> mux1/2
  in5/1 -> mux1/3
  in7/1 -> mux1/4
  rd_2/1 -> Serializer_Subnetwork1/2(in1)
  in9/1 -> mux1/5
  in11/1 -> mux1/6
  in15/1 -> mux1/8
  in39/1 -> mux1/20
  in19/1 -> mux1/10
  in27/1 -> mux1/14
  in21/1 -> mux1/11
  in29/1 -> mux1/15
  rd_7/1 -> dot_product1_bypass/2(in1)
  in35/1 -> mux1/18
  mux/1 -> Serializer_Subnetwork/1(in0)
  counter/1(out0) -> Serializer_Subnetwork/2(in1), rd_2/1
  mux1/1 -> rd_1/1
  Serializer_Subnetwork/1(out0) -> dot_product_7/1(in1)
  rd_1/1 -> Serializer_Subnetwork1/1(in0)
  rd_5/1 -> tappedDelay/Enable
  demux/17 -> out16/1
  Serializer_Subnetwork1/1(out0) -> dot_product_7/2(in2)
  dot_product_7/1(out1) -> rd_6/1, tappedDelay/1(in0)
  demux/3 -> out2/1
  demux/1 -> out0/1
  demux/4 -> out3/1
  demux/5 -> out4/1
  demux/6 -> out5/1
  demux/7 -> out6/1
  demux/8 -> out7/1
  demux/10 -> out9/1
  demux/11 -> out10/1
  demux/12 -> out11/1
  demux/13 -> out12/1
  demux/14 -> out13/1
  demux/15 -> out14/1
  demux/16 -> out15/1
  demux/18 -> out17/1
  demux/19 -> out18/1
  dot_product1_bypass/1(out0) -> out19/1

== system gm_HDL_pfc_gold_fi_og/simscape_system/simscape_system/HDL Subsystem/streaming_partition_streamed/Serializer_Subnetwork ==
  in0 : Inport  OutDataTypeStr=fixdt(1, 25, 13)  PortDimensions=[7]  SampleTime=1.0465724751439e-08
  in1 : Inport  Port=2  OutDataTypeStr=fixdt(0, 3, 0)  SampleTime=1.0465724751439e-08
  ratechange_splitcomp : Demux  Outputs=7
  splitcomp_multiport : MultiPortSwitch  DataPortOrder=Zero-based contiguous  Inputs=7  DiagnosticForDefault=None  zeroidx=on  OutDataTypeStr=fixdt(1, 25, 13)  SampleTime=1.0465724751439e-08  SaturateOnIntegerOverflow=off  InputSameDT=off
  out0 : Outport  OutDataTypeStr=fixdt(1, 25, 13)  SampleTime=1.0465724751439e-08
  wires:
  in0/1 -> ratechange_splitcomp/1
  ratechange_splitcomp/6 -> splitcomp_multiport/7
  in1/1 -> splitcomp_multiport/1
  ratechange_splitcomp/2 -> splitcomp_multiport/3
  ratechange_splitcomp/1 -> splitcomp_multiport/2
  ratechange_splitcomp/5 -> splitcomp_multiport/6
  ratechange_splitcomp/4 -> splitcomp_multiport/5
  ratechange_splitcomp/3 -> splitcomp_multiport/4
  ratechange_splitcomp/7 -> splitcomp_multiport/8
  splitcomp_multiport/1 -> out0/1

== system gm_HDL_pfc_gold_fi_og/simscape_system/simscape_system/HDL Subsystem/streaming_partition_streamed/Serializer_Subnetwork1 ==
  in0 : Inport  OutDataTypeStr=fixdt(1, 25, 13)  PortDimensions=[7]  SampleTime=1.0465724751439e-08
  in1 : Inport  Port=2  OutDataTypeStr=fixdt(0, 3, 0)  SampleTime=1.0465724751439e-08
  ratechange_splitcomp : Demux  Outputs=7
  splitcomp_multiport : MultiPortSwitch  DataPortOrder=Zero-based contiguous  Inputs=7  DiagnosticForDefault=None  zeroidx=on  OutDataTypeStr=fixdt(1, 25, 13)  SampleTime=1.0465724751439e-08  SaturateOnIntegerOverflow=off  InputSameDT=off
  out0 : Outport  OutDataTypeStr=fixdt(1, 25, 13)  SampleTime=1.0465724751439e-08
  wires:
  ratechange_splitcomp/1 -> splitcomp_multiport/2
  in0/1 -> ratechange_splitcomp/1
  in1/1 -> splitcomp_multiport/1
  ratechange_splitcomp/3 -> splitcomp_multiport/4
  ratechange_splitcomp/2 -> splitcomp_multiport/3
  ratechange_splitcomp/6 -> splitcomp_multiport/7
  ratechange_splitcomp/4 -> splitcomp_multiport/5
  splitcomp_multiport/1 -> out0/1
  ratechange_splitcomp/5 -> splitcomp_multiport/6
  ratechange_splitcomp/7 -> splitcomp_multiport/8

== system gm_HDL_pfc_gold_fi_og/simscape_system/simscape_system/HDL Subsystem/streaming_partition_streamed/counter ==
  globalSchedule : EnablePort  OutDataTypeStr=boolean
  ctr_0_6 : hdlsllib/Sources/HDL Counter  CountType=Count limited  CountInit=double(0)  CountStep=double(1)  CountMax=double(6)  CountFromType=Initial value  CountFrom=double(0)  CountResetPort=off  CountLoadPort=off  CountEnbPort=off  CountDirPort=off  CountHitOutputPort=off  CountDataType=Unsigned  CountWordLen=3  CountFracLen=0  CountSampTime=1.0465724751439e-08
  out0 : Outport  OutDataTypeStr=fixdt(0, 3, 0)  SampleTime=1.0465724751439e-08  InitialOutput=0
  wires:
  ctr_0_6/1 -> out0/1

== system gm_HDL_pfc_gold_fi_og/simscape_system/simscape_system/HDL Subsystem/streaming_partition_streamed/delayInSignal_bypass ==
  in0 : Inport  OutDataTypeStr=fixdt(1, 25, 13)  SampleTime=1.0465724751439e-08
  in1 : Inport  Port=2  OutDataTypeStr=boolean  SampleTime=1.0465724751439e-08
  delayInSignal_enb : Switch  Criteria=u2 ~= 0  Threshold=double(0)  OutDataTypeStr=fixdt(1, 25, 13)  SampleTime=1.0465724751439e-08  SaturateOnIntegerOverflow=off  InputSameDT=off
  delayInSignal_state : Delay  DelayLength=double(1)  InitialCondition=0  SampleTime=1.0465724751439e-08
  out0 : Outport  OutDataTypeStr=fixdt(1, 25, 13)  SampleTime=1.0465724751439e-08
  wires:
  in0/1 -> delayInSignal_enb/1
  in1/1 -> delayInSignal_enb/2
  delayInSignal_state/1 -> delayInSignal_enb/3
  delayInSignal_enb/1 -> delayInSignal_state/1, out0/1

== system gm_HDL_pfc_gold_fi_og/simscape_system/simscape_system/HDL Subsystem/streaming_partition_streamed/tappedDelay ==
  in0 : Inport  OutDataTypeStr=fixdt(1, 25, 13)  SampleTime=1.0465724751439e-08
  globalSchedule : EnablePort  OutDataTypeStr=boolean
  StateControl : StateControl  StateControl=Synchronous
  tapped_delay : simulink/Discrete/Tapped Delay  vinit=0  samptime=-1  NumDelays=double(6)  DelayOrder=Oldest  includeCurrent=off
  out0 : Outport  OutDataTypeStr=fixdt(1, 25, 13)  PortDimensions=[6]  SampleTime=1.0465724751439e-08  InitialOutput=0
  wires:
  in0/1 -> tapped_delay/1
  tapped_delay/1 -> out0/1

== system gm_HDL_pfc_gold_fi_og/simscape_system/simscape_system/HDL Subsystem/streaming_partition_streamed1/Serializer_Subnetwork ==
  in0 : Inport  OutDataTypeStr=fixdt(1, 25, 13)  PortDimensions=[7]  SampleTime=1.0465724751439e-08
  in1 : Inport  Port=2  OutDataTypeStr=fixdt(0, 3, 0)  SampleTime=1.0465724751439e-08
  ratechange_splitcomp : Demux  Outputs=7
  splitcomp_multiport : MultiPortSwitch  DataPortOrder=Zero-based contiguous  Inputs=7  DiagnosticForDefault=None  zeroidx=on  OutDataTypeStr=fixdt(1, 25, 13)  SampleTime=1.0465724751439e-08  SaturateOnIntegerOverflow=off  InputSameDT=off
  out0 : Outport  OutDataTypeStr=fixdt(1, 25, 13)  SampleTime=1.0465724751439e-08
  wires:
  in0/1 -> ratechange_splitcomp/1
  ratechange_splitcomp/3 -> splitcomp_multiport/4
  in1/1 -> splitcomp_multiport/1
  ratechange_splitcomp/2 -> splitcomp_multiport/3
  ratechange_splitcomp/1 -> splitcomp_multiport/2
  ratechange_splitcomp/4 -> splitcomp_multiport/5
  ratechange_splitcomp/5 -> splitcomp_multiport/6
  ratechange_splitcomp/6 -> splitcomp_multiport/7
  ratechange_splitcomp/7 -> splitcomp_multiport/8
  splitcomp_multiport/1 -> out0/1

== system gm_HDL_pfc_gold_fi_og/simscape_system/simscape_system/HDL Subsystem/streaming_partition_streamed1/Serializer_Subnetwork1 ==
  in0 : Inport  OutDataTypeStr=fixdt(1, 25, 13)  PortDimensions=[7]  SampleTime=1.0465724751439e-08
  in1 : Inport  Port=2  OutDataTypeStr=fixdt(0, 3, 0)  SampleTime=1.0465724751439e-08
  ratechange_splitcomp : Demux  Outputs=7
  splitcomp_multiport : MultiPortSwitch  DataPortOrder=Zero-based contiguous  Inputs=7  DiagnosticForDefault=None  zeroidx=on  OutDataTypeStr=fixdt(1, 25, 13)  SampleTime=1.0465724751439e-08  SaturateOnIntegerOverflow=off  InputSameDT=off
  out0 : Outport  OutDataTypeStr=fixdt(1, 25, 13)  SampleTime=1.0465724751439e-08
  wires:
  in0/1 -> ratechange_splitcomp/1
  in1/1 -> splitcomp_multiport/1
  ratechange_splitcomp/1 -> splitcomp_multiport/2
  ratechange_splitcomp/2 -> splitcomp_multiport/3
  ratechange_splitcomp/6 -> splitcomp_multiport/7
  ratechange_splitcomp/5 -> splitcomp_multiport/6
  ratechange_splitcomp/4 -> splitcomp_multiport/5
  ratechange_splitcomp/3 -> splitcomp_multiport/4
  ratechange_splitcomp/7 -> splitcomp_multiport/8
  splitcomp_multiport/1 -> out0/1

== system gm_HDL_pfc_gold_fi_og/simscape_system/simscape_system/HDL Subsystem/streaming_partition_streamed1/counter ==
  globalSchedule : EnablePort  OutDataTypeStr=boolean
  ctr_0_6 : hdlsllib/Sources/HDL Counter  CountType=Count limited  CountInit=double(0)  CountStep=double(1)  CountMax=double(6)  CountFromType=Initial value  CountFrom=double(0)  CountResetPort=off  CountLoadPort=off  CountEnbPort=off  CountDirPort=off  CountHitOutputPort=off  CountDataType=Unsigned  CountWordLen=3  CountFracLen=0  CountSampTime=1.0465724751439e-08
  out0 : Outport  OutDataTypeStr=fixdt(0, 3, 0)  SampleTime=1.0465724751439e-08  InitialOutput=0
  wires:
  ctr_0_6/1 -> out0/1

== system gm_HDL_pfc_gold_fi_og/simscape_system/simscape_system/HDL Subsystem/streaming_partition_streamed1/delayOutSignal_bypass ==
  in0 : Inport  OutDataTypeStr=fixdt(1, 25, 13)  SampleTime=1.0465724751439e-08
  in1 : Inport  Port=2  OutDataTypeStr=boolean  SampleTime=1.0465724751439e-08
  delayOutSignal_enb : Switch  Criteria=u2 ~= 0  Threshold=double(0)  OutDataTypeStr=fixdt(1, 25, 13)  SampleTime=1.0465724751439e-08  SaturateOnIntegerOverflow=off  InputSameDT=off
  delayOutSignal_state : Delay  DelayLength=double(1)  InitialCondition=0  SampleTime=1.0465724751439e-08
  out0 : Outport  OutDataTypeStr=fixdt(1, 25, 13)  SampleTime=1.0465724751439e-08
  wires:
  in1/1 -> delayOutSignal_enb/2
  in0/1 -> delayOutSignal_enb/1
  delayOutSignal_state/1 -> delayOutSignal_enb/3
  delayOutSignal_enb/1 -> delayOutSignal_state/1, out0/1

== system gm_HDL_pfc_gold_fi_og/simscape_system/simscape_system/HDL Subsystem/streaming_partition_streamed1/tappedDelay ==
  in0 : Inport  OutDataTypeStr=fixdt(1, 25, 13)  SampleTime=1.0465724751439e-08
  globalSchedule : EnablePort  OutDataTypeStr=boolean
  StateControl : StateControl  StateControl=Synchronous
  tapped_delay : simulink/Discrete/Tapped Delay  vinit=0  samptime=-1  NumDelays=double(6)  DelayOrder=Oldest  includeCurrent=off
  out0 : Outport  OutDataTypeStr=fixdt(1, 25, 13)  PortDimensions=[6]  SampleTime=1.0465724751439e-08  InitialOutput=0
  wires:
  in0/1 -> tapped_delay/1
  tapped_delay/1 -> out0/1

== system gm_HDL_pfc_gold_fi_og/simscape_system/simscape_system/HDL Subsystem/Sparse Matrix-Vector Product/hNNewMatrixB_shared/Serializer_Subnetwork ==
  in0 : Inport  OutDataTypeStr=fixdt(1, 25, 31)  PortDimensions=[63]  SampleTime=1.0465724751439e-08
  in1 : Inport  Port=2  OutDataTypeStr=fixdt(0, 3, 0)  SampleTime=1.0465724751439e-08
  ratechange_splitcomp : Demux  Outputs=7
  splitcomp_multiport : MultiPortSwitch  DataPortOrder=Zero-based contiguous  Inputs=7  DiagnosticForDefault=None  zeroidx=on  OutDataTypeStr=fixdt(1, 25, 31)  SampleTime=1.0465724751439e-08  SaturateOnIntegerOverflow=off  InputSameDT=off
  out0 : Outport  OutDataTypeStr=fixdt(1, 25, 31)  PortDimensions=[9]  SampleTime=1.0465724751439e-08
  wires:
  ratechange_splitcomp/2 -> splitcomp_multiport/3
  in0/1 -> ratechange_splitcomp/1
  in1/1 -> splitcomp_multiport/1
  ratechange_splitcomp/4 -> splitcomp_multiport/5
  ratechange_splitcomp/1 -> splitcomp_multiport/2
  ratechange_splitcomp/6 -> splitcomp_multiport/7
  ratechange_splitcomp/3 -> splitcomp_multiport/4
  ratechange_splitcomp/5 -> splitcomp_multiport/6
  ratechange_splitcomp/7 -> splitcomp_multiport/8
  splitcomp_multiport/1 -> out0/1

== system gm_HDL_pfc_gold_fi_og/simscape_system/simscape_system/HDL Subsystem/Sparse Matrix-Vector Product/hNNewMatrixB_shared/Serializer_Subnetwork1 ==
  in0 : Inport  OutDataTypeStr=fixdt(1, 25, 13)  PortDimensions=[63]  SampleTime=1.0465724751439e-08
  in1 : Inport  Port=2  OutDataTypeStr=fixdt(0, 3, 0)  SampleTime=1.0465724751439e-08
  ratechange_splitcomp : Demux  Outputs=7
  splitcomp_multiport : MultiPortSwitch  DataPortOrder=Zero-based contiguous  Inputs=7  DiagnosticForDefault=None  zeroidx=on  OutDataTypeStr=fixdt(1, 25, 13)  SampleTime=1.0465724751439e-08  SaturateOnIntegerOverflow=off  InputSameDT=off
  out0 : Outport  OutDataTypeStr=fixdt(1, 25, 13)  PortDimensions=[9]  SampleTime=1.0465724751439e-08
  wires:
  in0/1 -> ratechange_splitcomp/1
  ratechange_splitcomp/3 -> splitcomp_multiport/4
  in1/1 -> splitcomp_multiport/1
  ratechange_splitcomp/1 -> splitcomp_multiport/2
  ratechange_splitcomp/5 -> splitcomp_multiport/6
  ratechange_splitcomp/2 -> splitcomp_multiport/3
  ratechange_splitcomp/4 -> splitcomp_multiport/5
  ratechange_splitcomp/6 -> splitcomp_multiport/7
  ratechange_splitcomp/7 -> splitcomp_multiport/8
  splitcomp_multiport/1 -> out0/1

== system gm_HDL_pfc_gold_fi_og/simscape_system/simscape_system/HDL Subsystem/Sparse Matrix-Vector Product/hNNewMatrixB_shared/counter ==
  globalSchedule : EnablePort  OutDataTypeStr=boolean
  ctr_0_6 : hdlsllib/Sources/HDL Counter  CountType=Count limited  CountInit=double(0)  CountStep=double(1)  CountMax=double(6)  CountFromType=Initial value  CountFrom=double(0)  CountResetPort=off  CountLoadPort=off  CountEnbPort=off  CountDirPort=off  CountHitOutputPort=off  CountDataType=Unsigned  CountWordLen=3  CountFracLen=0  CountSampTime=1.0465724751439e-08
  out0 : Outport  OutDataTypeStr=fixdt(0, 3, 0)  SampleTime=1.0465724751439e-08  InitialOutput=0
  wires:
  ctr_0_6/1 -> out0/1

== system gm_HDL_pfc_gold_fi_og/simscape_system/simscape_system/HDL Subsystem/Sparse Matrix-Vector Product/hNNewMatrixB_shared/dot_product1_bypass ==
  in0 : Inport  OutDataTypeStr=fixdt(1, 50, 44)  SampleTime=1.0465724751439e-08
  in1 : Inport  Port=2  OutDataTypeStr=boolean  SampleTime=1.0465724751439e-08
  dot_product1_enb : Switch  Criteria=u2 ~= 0  Threshold=double(0)  OutDataTypeStr=fixdt(1, 50, 44)  SampleTime=1.0465724751439e-08  SaturateOnIntegerOverflow=off  InputSameDT=off
  dot_product1_state : Delay  DelayLength=double(1)  InitialCondition=0  SampleTime=1.0465724751439e-08
  out0 : Outport  OutDataTypeStr=fixdt(1, 50, 44)  SampleTime=1.0465724751439e-08
  wires:
  in0/1 -> dot_product1_enb/1
  in1/1 -> dot_product1_enb/2
  dot_product1_state/1 -> dot_product1_enb/3
  dot_product1_enb/1 -> out0/1, dot_product1_state/1

== system gm_HDL_pfc_gold_fi_og/simscape_system/simscape_system/HDL Subsystem/Sparse Matrix-Vector Product/hNNewMatrixB_shared/dot_product_9 ==
  in1 : Inport  OutDataTypeStr=fixdt(1, 25, 31)  PortDimensions=[9]  SampleTime=1.0465724751439e-08
  in2 : Inport  Port=2  OutDataTypeStr=fixdt(1, 25, 13)  PortDimensions=[9]  SampleTime=1.0465724751439e-08
  HwModeRegister : Delay  DelayLength=double(1)  InitialCondition=0  SampleTime=1.0465724751439e-08
  HwModeRegister1 : Delay  DelayLength=double(1)  InitialCondition=0  SampleTime=1.0465724751439e-08
  PipelineRegister : Delay  DelayLength=double(1)  InitialCondition=0  SampleTime=1.0465724751439e-08
  adder{,1..7} (8 alike) : Sum  OutDataTypeStr=fixdt(1, 50, 44)  SampleTime=1.0465724751439e-08
  mul_out1_8_wire : hdlmdlgenlib/Buffer
  multiplier : Product  Inputs=**  OutDataTypeStr=fixdt(1, 50, 44)  SampleTime=1.0465724751439e-08
  rd_0 : Delay  DelayLength=double(6)  InitialCondition=0  SampleTime=1.0465724751439e-08
  rd_{1..5} (5 alike) : Delay  DelayLength=double(1)  InitialCondition=0  SampleTime=1.0465724751439e-08
  rd_6 : Delay  DelayLength=double(2)  InitialCondition=0  SampleTime=1.0465724751439e-08
  sum_stage1_5_wire : hdlmdlgenlib/Buffer
  sum_stage2_3_wire : hdlmdlgenlib/Buffer
  sum_stage4_1_wire : hdlmdlgenlib/Buffer
  t : Demux  Outputs=9
  out1 : Outport  OutDataTypeStr=fixdt(1, 50, 44)  SampleTime=1.0465724751439e-08
  wires:
  in1/1 -> rd_0/1
  multiplier/1 -> PipelineRegister/1
  in2/1 -> HwModeRegister1/1
  t/3 -> adder1/1
  rd_0/1 -> HwModeRegister/1
  t/5 -> adder2/1
  t/1 -> adder/1
  t/9 -> mul_out1_8_wire/1
  PipelineRegister/1 -> t/1
  t/8 -> adder3/2
  HwModeRegister/1 -> multiplier/1
  mul_out1_8_wire/1 -> sum_stage1_5_wire/1
  HwModeRegister1/1 -> multiplier/2
  rd_4/1 -> adder5/2
  t/4 -> adder1/2
  t/2 -> adder/2
  t/6 -> adder2/2
  t/7 -> adder3/1
  adder/1 -> rd_1/1
  adder1/1 -> rd_2/1
  adder2/1 -> rd_3/1
  adder3/1 -> rd_4/1
  rd_1/1 -> adder4/1
  rd_2/1 -> adder4/2
  rd_3/1 -> adder5/1
  sum_stage1_5_wire/1 -> sum_stage2_3_wire/1
  adder4/1 -> adder6/1
  adder5/1 -> adder6/2
  sum_stage2_3_wire/1 -> rd_6/1
  adder6/1 -> rd_5/1
  rd_5/1 -> adder7/1
  rd_6/1 -> adder7/2
  adder7/1 -> sum_stage4_1_wire/1
  sum_stage4_1_wire/1 -> out1/1

== system gm_HDL_pfc_gold_fi_og/simscape_system/simscape_system/HDL Subsystem/Sparse Matrix-Vector Product/hNNewMatrixB_shared/tappedDelay ==
  in0 : Inport  OutDataTypeStr=fixdt(1, 50, 44)  SampleTime=1.0465724751439e-08
  globalSchedule : EnablePort  OutDataTypeStr=boolean
  StateControl : StateControl  StateControl=Synchronous
  tappedDelay : simulink/Discrete/Tapped Delay  vinit=0  samptime=-1  NumDelays=double(6)  DelayOrder=Oldest  includeCurrent=off
  out0 : Outport  OutDataTypeStr=fixdt(1, 50, 44)  PortDimensions=[6]  SampleTime=1.0465724751439e-08  InitialOutput=0
  wires:
  in0/1 -> tappedDelay/1
  tappedDelay/1 -> out0/1

== system gm_HDL_pfc_gold_fi_og/simscape_system/simscape_system/HDL Subsystem/Sparse Matrix-Vector Product1/hNNewMatrixA_shared/Serializer_Subnetwork ==
  in0 : Inport  OutDataTypeStr=fixdt(1, 25, 24)  PortDimensions=[42]  SampleTime=1.0465724751439e-08
  in1 : Inport  Port=2  OutDataTypeStr=fixdt(0, 3, 0)  SampleTime=1.0465724751439e-08
  ratechange_splitcomp : Demux  Outputs=7
  splitcomp_multiport : MultiPortSwitch  DataPortOrder=Zero-based contiguous  Inputs=7  DiagnosticForDefault=None  zeroidx=on  OutDataTypeStr=fixdt(1, 25, 24)  SampleTime=1.0465724751439e-08  SaturateOnIntegerOverflow=off  InputSameDT=off
  out0 : Outport  OutDataTypeStr=fixdt(1, 25, 24)  PortDimensions=[6]  SampleTime=1.0465724751439e-08
  wires:
  ratechange_splitcomp/4 -> splitcomp_multiport/5
  in0/1 -> ratechange_splitcomp/1
  in1/1 -> splitcomp_multiport/1
  ratechange_splitcomp/1 -> splitcomp_multiport/2
  ratechange_splitcomp/3 -> splitcomp_multiport/4
  ratechange_splitcomp/2 -> splitcomp_multiport/3
  ratechange_splitcomp/5 -> splitcomp_multiport/6
  ratechange_splitcomp/6 -> splitcomp_multiport/7
  ratechange_splitcomp/7 -> splitcomp_multiport/8
  splitcomp_multiport/1 -> out0/1

== system gm_HDL_pfc_gold_fi_og/simscape_system/simscape_system/HDL Subsystem/Sparse Matrix-Vector Product1/hNNewMatrixA_shared/Serializer_Subnetwork1 ==
  in0 : Inport  OutDataTypeStr=fixdt(1, 25, 13)  PortDimensions=[42]  SampleTime=1.0465724751439e-08
  in1 : Inport  Port=2  OutDataTypeStr=fixdt(0, 3, 0)  SampleTime=1.0465724751439e-08
  ratechange_splitcomp : Demux  Outputs=7
  splitcomp_multiport : MultiPortSwitch  DataPortOrder=Zero-based contiguous  Inputs=7  DiagnosticForDefault=None  zeroidx=on  OutDataTypeStr=fixdt(1, 25, 13)  SampleTime=1.0465724751439e-08  SaturateOnIntegerOverflow=off  InputSameDT=off
  out0 : Outport  OutDataTypeStr=fixdt(1, 25, 13)  PortDimensions=[6]  SampleTime=1.0465724751439e-08
  wires:
  in0/1 -> ratechange_splitcomp/1
  in1/1 -> splitcomp_multiport/1
  ratechange_splitcomp/1 -> splitcomp_multiport/2
  ratechange_splitcomp/3 -> splitcomp_multiport/4
  ratechange_splitcomp/5 -> splitcomp_multiport/6
  ratechange_splitcomp/2 -> splitcomp_multiport/3
  ratechange_splitcomp/4 -> splitcomp_multiport/5
  ratechange_splitcomp/6 -> splitcomp_multiport/7
  splitcomp_multiport/1 -> out0/1
  ratechange_splitcomp/7 -> splitcomp_multiport/8

== system gm_HDL_pfc_gold_fi_og/simscape_system/simscape_system/HDL Subsystem/Sparse Matrix-Vector Product1/hNNewMatrixA_shared/counter ==
  globalSchedule : EnablePort  OutDataTypeStr=boolean
  ctr_0_6 : hdlsllib/Sources/HDL Counter  CountType=Count limited  CountInit=double(0)  CountStep=double(1)  CountMax=double(6)  CountFromType=Initial value  CountFrom=double(0)  CountResetPort=off  CountLoadPort=off  CountEnbPort=off  CountDirPort=off  CountHitOutputPort=off  CountDataType=Unsigned  CountWordLen=3  CountFracLen=0  CountSampTime=1.0465724751439e-08
  out0 : Outport  OutDataTypeStr=fixdt(0, 3, 0)  SampleTime=1.0465724751439e-08  InitialOutput=0
  wires:
  ctr_0_6/1 -> out0/1
